simulink model "fuzzy_no_load_no_delay"  (Simulink 9.3)
settings: Solver=FixedStepAuto  StartTime=0.0  StopTime=25  FixedStep=0.01  RelTol=1e-3
undefined symbols (not defined in the file or in its folder): DiscIntNeverNeededParam
libraries: fuzblock x3, simulink x1
settings Model: Creator=TDNhon  LastModifiedBy=minhk
settings DataIOCC: SaveFormat=Dataset  SignalLoggingSaveFormat=Dataset
settings OptimizationCC: LifeSpan=auto
settings DebuggingCC: UnderspecifiedInitializationDetection=Simplified  MergeDetectMultiDrivingBlocksExec=error  FcnCallInpInsideContextMsg=error  PregeneratedLibrarySubsystemCodeDiagnostic=none  SFUnexpectedBacktrackingDiag=error  SFNoUnconditionalDefaultTransitionDiag=error  SFExecutionAtInitializationDiag=warning
settings HardwareCC: ProdBitPerPointer=64  ProdBitPerSizeT=64  ProdBitPerPtrDiffT=64  ProdLargestAtomicFloat=Float  ProdIntDivRoundTo=Zero  ProdEndianess=LittleEndian  ProdWordSize=64  ProdHWDeviceType=Intel->x86-64 (Windows64)
settings ModelReferenceCC: PropagateSignalLabelsOutOfModel=on
settings CodeAppCC: StateflowObjectComments=off
settings GRTTargetCC: TargetLangStandard=C99 (ISO)  CombineOutputUpdateFcns=on  GRTInterface=off
settings ConfigComp: CovMetricSettings=dwe  CovHtmlReporting=off  CovSaveCumulativeToWorkspaceVar=off  CovSaveSingleToWorkspaceVar=off  CovExternalEMLEnable=on

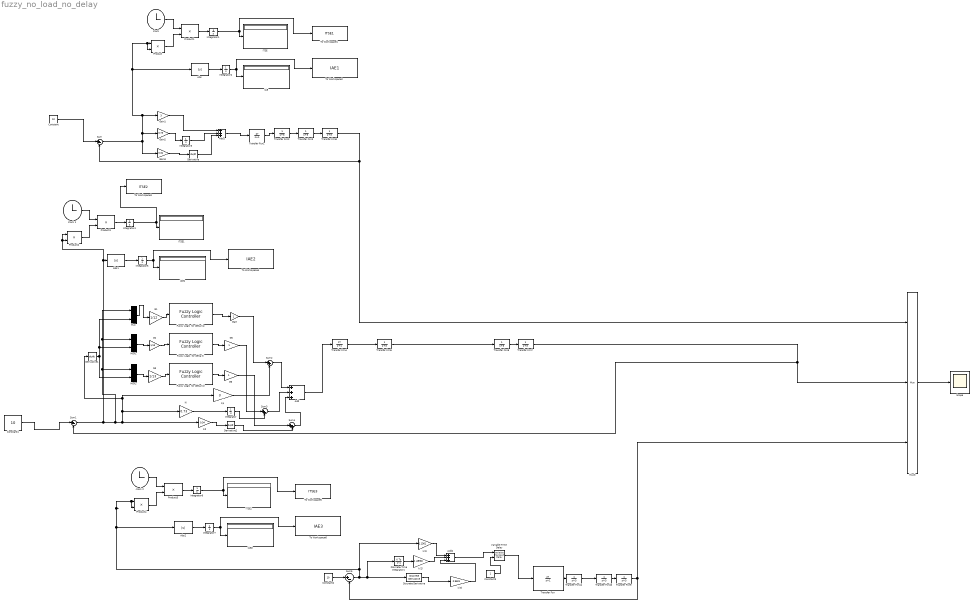
== system fuzzy_no_load_no_delay ==
  Abs : Abs
  Abs1 : Abs
  Abs2 : Abs
  Add : Sum  Inputs=+++
  Add1 : Sum  Inputs=+++
  Add2 : Sum  Inputs=+++
  Constant : Constant  Value=10
  Constant1 : Constant  Value=10
  Constant2 : Constant  Value=10
  Constant3 : Constant
  Derivative : Derivative
  Derivative1 : Derivative
  Derivative2 : Derivative
  Discrete Derivative : simulink/Discrete/Discrete Derivative  gainval=1.0  ICPrevScaledInput=0.0  OutMin=[]  OutMax=[]  OutDataType=fixdt(1, 16)  OutScaling=2^-10  DoSatur=off
  Discrete-Time Integrator1 : DiscreteIntegrator  SampleTime=-1  ICPrevOutput=DiscIntNeverNeededParam  ICPrevScaledInput=DiscIntNeverNeededParam
  Fuzzy Logic  for delta Kd : fuzblock/Fuzzy Logic  Controller  FIS='fuzzy_delta_Kd.fis'  OutputSampleNumber=101  DataType=double  FuzzifiedInputs=off  RuleFiringStrengths=off  RuleOutputs=off  AggregatedOutputs=off  SimulateUsing=Interpreted execution  OutOfRangeInputValueMessage=warning  NoRuleFiredMessage=warning  EmptyOutputFuzzySetMessage=warning
  "Fuzzy Logic  for delta Ki " : fuzblock/Fuzzy Logic  Controller  FIS='fuzzy_delta_Ki.fis'  OutputSampleNumber=101  DataType=double  FuzzifiedInputs=off  RuleFiringStrengths=off  RuleOutputs=off  AggregatedOutputs=off  SimulateUsing=Interpreted execution  OutOfRangeInputValueMessage=warning  NoRuleFiredMessage=warning  EmptyOutputFuzzySetMessage=warning
  "Fuzzy Logic  for delta Kp " : fuzblock/Fuzzy Logic  Controller  FIS='fuzzy_delta_Kp.fis'  OutputSampleNumber=101  DataType=double  FuzzifiedInputs=off  RuleFiringStrengths=off  RuleOutputs=off  AggregatedOutputs=off  SimulateUsing=Interpreted execution  OutOfRangeInputValueMessage=warning  NoRuleFiredMessage=warning  EmptyOutputFuzzySetMessage=warning
  G1 : Gain  Gain=1/12
  G2 : Gain  Gain=1/13
  G3 : Gain  Gain=1/13
  G5 : Gain
  "G6 " : Gain
  Gain : Gain
  Gain1 : Gain  Gain=3
  Gain2 : Gain  Gain=0.73
  Gain3 : Gain  Gain=0.34
  IAE : Display
  IAE1 : Display
  IAE2 : Display
  ITSE : Display
  ITSE1 : Display
  ITSE2 : Display
  Integrator{,1..7} (8 alike) : Integrator
  Kd : Gain  Gain=0.34
  Ki : Gain  Gain=0.73
  "Kp " : Gain  Gain=3
  Mux : Mux  Inputs=2
  Mux1 : Mux  Inputs=2
  Mux2 : Mux  Inputs=2
  Mux3 : Mux  Inputs=3
  Product{,1..5} (6 alike) : Product
  Scope : Scope
  Sum : Sum  Inputs=|+-
  Sum1 : Sum  Inputs=|+-
  Sum2 : Sum  Inputs=|++
  Sum3 : Sum  Inputs=|++
  Sum4 : Sum  Inputs=|++
  Sum5 : Sum  Inputs=|+-
  To Workspace1 : ToWorkspace  VariableName=ITSE1  SampleTime=-1
  To Workspace2 : ToWorkspace  VariableName=IAE1  SampleTime=-1
  To Workspace3 : ToWorkspace  VariableName=ITSE2  SampleTime=-1
  To Workspace4 : ToWorkspace  VariableName=IAE2  SampleTime=-1
  To Workspace5 : ToWorkspace  VariableName=ITSE3  SampleTime=-1
  To Workspace6 : ToWorkspace  VariableName=IAE3  SampleTime=-1
  Transfer Fcn : TransferFcn  Numerator=[27]  Denominator=[1 1]
  Transfer Fcn1 : TransferFcn  Numerator=[27]  Denominator=[1 1]
  Transfer Fcn{2..3,5..11} (9 alike) : TransferFcn  Denominator=[1 3]
  Transfer Fcn4 : TransferFcn  Numerator=[27]  Denominator=[1 1]
  Variable Time Delay : VariableTransportDelay  MaximumDelay=10
  "clock " : Clock
  clock 1 : Clock
  clock 2 : Clock
  k(1) : Gain  Gain=1.1361
  k(2) : Gain  Gain=0.4990
  k(3) : Gain  Gain=0.9601
  wires:
  Sum1/1 -> Product2/1, Product2/2, Abs1/1, Mux2/1, Mux/1, Mux1/1, "Kp "/1, Derivative1/1, Ki/1, Kd/1
  "Fuzzy Logic  for delta Kp "/1 -> Gain/1
  Ki/1 -> Integrator/1
  Sum2/1 -> Add/1
  "G6 "/1 -> Sum4/1
  G2/1 -> "Fuzzy Logic  for delta Ki "/1
  Transfer Fcn7/1 -> Mux3/2, Sum1/2
  Mux1/1 -> G2/1
  Fuzzy Logic  for delta Kd/1 -> "G6 "/1
  G1/1 -> "Fuzzy Logic  for delta Kp "/1
  Kd/1 -> Derivative2/1
  Derivative2/1 -> Sum4/2
  Transfer Fcn6/1 -> Transfer Fcn7/1
  Integrator/1 -> Sum3/2
  G5/1 -> Sum3/1
  "Fuzzy Logic  for delta Ki "/1 -> G5/1
  G3/1 -> Fuzzy Logic  for delta Kd/1
  "Kp "/1 -> Sum2/2
  Transfer Fcn5/1 -> Transfer Fcn6/1
  Mux/1 -> G1/1
  Mux2/1 -> G3/1
  Transfer Fcn4/1 -> Transfer Fcn5/1
  Derivative1/1 -> Mux2/2, Mux1/2, Mux/2
  Sum3/1 -> Add/2
  Sum4/1 -> Add/3
  Gain/1 -> Sum2/1
  Gain2/1 -> Integrator3/1
  Derivative/1 -> Add1/3
  Integrator3/1 -> Add1/2
  Transfer Fcn8/1 -> Mux3/1, Sum/2
  Transfer Fcn1/1 -> Transfer Fcn2/1
  Gain1/1 -> Add1/1
  Constant/1 -> Sum/1
  Transfer Fcn2/1 -> Transfer Fcn3/1
  Gain3/1 -> Derivative/1
  Transfer Fcn3/1 -> Transfer Fcn8/1
  k(3)/1 -> Add2/3
  Transfer Fcn/1 -> Transfer Fcn11/1
  Transfer Fcn11/1 -> Transfer Fcn10/1
  Variable Time Delay/1 -> Transfer Fcn/1
  Add2/1 -> Variable Time Delay/1
  Constant2/1 -> Sum5/1
  k(2)/1 -> Add2/2
  Discrete-Time Integrator1/1 -> k(2)/1
  Transfer Fcn10/1 -> Transfer Fcn9/1
  k(1)/1 -> Add2/1
  Constant3/1 -> Variable Time Delay/2
  Discrete Derivative/1 -> k(3)/1
  Add/1 -> Transfer Fcn4/1
  Add1/1 -> Transfer Fcn1/1
  Mux3/1 -> Scope/1
  Transfer Fcn9/1 -> Mux3/3, Sum5/2
  Integrator1/1 -> To Workspace1/1, ITSE/1
  "clock "/1 -> Product1/1
  Sum/1 -> Abs/1, Product/2, Product/1, Gain1/1, Gain2/1, Gain3/1
  Abs/1 -> Integrator2/1
  Integrator2/1 -> To Workspace2/1, IAE/1
  Product1/1 -> Integrator1/1
  Product/1 -> Product1/2
  Integrator4/1 -> To Workspace3/1, ITSE1/1
  clock 1/1 -> Product3/1
  Constant1/1 -> Sum1/1
  Abs1/1 -> Integrator5/1
  Integrator5/1 -> To Workspace4/1, IAE1/1
  Product3/1 -> Integrator4/1
  Product2/1 -> Product3/2
  Integrator6/1 -> To Workspace5/1, ITSE2/1
  clock 2/1 -> Product5/1
  Sum5/1 -> k(1)/1, Abs2/1, Product4/2, Product4/1, Discrete Derivative/1, Discrete-Time Integrator1/1
  Abs2/1 -> Integrator7/1
  Integrator7/1 -> To Workspace6/1, IAE2/1
  Product5/1 -> Integrator6/1
  Product4/1 -> Product5/2
